simulink model "mavsim_chap10_6DOF"  (R2020b)
settings: Solver=ode15s  StartTime=0.0  StopTime=400  RelTol=1e-3  EnableMultiTasking=on
InitFcn:
  | param_chap10
undefined symbols (not defined in the file or in its folder): autopilot, drawPathError, Earth, forces_moments, js_decode_landing, js_encode_landing, P, path_follow, path_manager_chap10, sigbuilder_block, true_states, WGS84
libraries: simulink x7, simulink_extras x7, pid_lib x7, aerolibfltsims x2, instrumentlib x2, shared6dof x1, aerolibasang x1, aerolibtransform2 x1, aerolibanimutils x1, dspnetwork x1
(part 1 of 2)
settings Model: Creator=beard  LastModifiedBy=jk
settings DataIOCC: LimitDataPoints=on  SaveFormat=Array  SignalLoggingSaveFormat=ModelDataLogs  ReturnWorkspaceOutputs=off
settings OptimizationCC: ExpressionDepthLimit=2147483647  InitFltsAndDblsToZero=on  LifeSpan=inf
settings DebuggingCC: UnderspecifiedInitializationDetection=Classic  MergeDetectMultiDrivingBlocksExec=none  SolverPrmCheckMsg=warning  FcnCallInpInsideContextMsg=warning  StateNameClashWarn=warning  SFUnexpectedBacktrackingDiag=warning  SFNoUnconditionalDefaultTransitionDiag=warning  SFExecutionAtInitializationDiag=none  ArithmeticOperatorsInVariantConditions=warning
settings HardwareCC: ProdBitPerPointer=32  ProdBitPerSizeT=32  ProdBitPerPtrDiffT=32  ProdLargestAtomicFloat=None  ProdIntDivRoundTo=Undefined  ProdEndianess=Unspecified  ProdWordSize=32  ProdHWDeviceType=32-bit Generic
settings ModelReferenceCC: PropagateSignalLabelsOutOfModel=off
settings SFSimCC: SimUseLocalCustomCode=off  SimParseCustomCode=off  CustomCodeUndefinedFunction=UseInterfaceOnly
settings RTWCC: RTWUseLocalCustomCode=off
settings CodeAppCC: StateflowObjectComments=on
settings GRTTargetCC: TargetLangStandard=C89/C90 (ANSI)  CombineOutputUpdateFcns=off  GRTInterface=on
settings ConfigComp: CovMetricSettings=dw  CovSaveCumulativeToWorkspaceVar=on  CovSaveSingleToWorkspaceVar=on  CovExternalEMLEnable=off  CovSFcnEnable=off

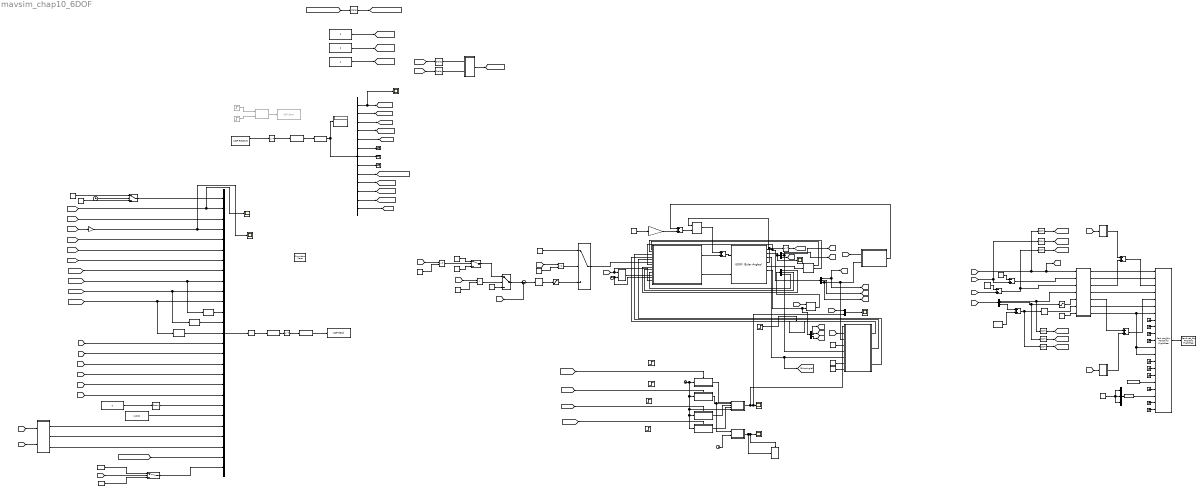
== system mavsim_chap10_6DOF ==
  note: 接受到来自航母终止盘旋指令
  note: 接受到来自航母的盘旋指令
  note: 开始着舰
  note: 开始降落
  note: 通过UDP接收数据，暂时通过自己创造Json的形式来测试是否正常接收，联调的时候将此区域内的发送部分删除只保留接收
  note: 发送部分用于测试使用
  note: 偏差XYZ
  note: 推力控制
  6DOF (Euler Angles) : shared6dof/6DOF (Euler Angles)  units=Metric (MKS)  mtype=Fixed  rep=Euler Angles  xme_0=[-5226.5 0 -600]  Vm_0=[80*cosd(-0) 0 80*sind(-0)]  eul_0=[0 -0*pi/180 0]  pm_0=[0 0 0]  mass_0=11000  mass_e=0.5  mass_f=2.0  inertia=[1000,0,0;0,2000,0;0,0,1000]  inertia_e=eye(3)  inertia_f=2*eye(3)  k_quat=1.0  vre_flag=on  abi_flag=off  aMode=0  xme_statename=''  Vm_statename=''  eul_statename=''  quat_statename=''  pm_statename=''  mass_statename=''
      settings: SourceProductBaseCode=AE,PW,MT,UV,VE,VP
  Add{,1,3..4,7} (5 alike) : Sum
  Add2 : Sum  Inputs=-+
  Add5 : Sum  Inputs=-+
  Clock{,1..3} (4 alike) : Clock
  Constant{,1,10,12,14,19..20} (7 alike) : Constant  Value=0
  Constant11 : Constant  Value=11000
  Constant13 : Constant  Value=2
  Constant{15..18,22} (5 alike) : Constant
  Constant2 : Constant  Value=-0.06
  Constant21 : Constant  Value=-40
  Constant3 : Constant  Value=3  OutDataTypeStr=uint32
  Constant4 : Constant  Value=-700
  Constant5 : Constant  Value=-300
  Constant6 : Constant  Value=80
  Constant7 : Constant  Value=120
  Constant8 : Constant  Value=70
  Constant9 : Constant  Value=-30
  Data Type Conversion : DataTypeConversion  OutDataTypeStr=double
  Data Type Conversion1 : DataTypeConversion  OutDataTypeStr=uint8
  Data Type Conversion2 : DataTypeConversion  OutDataTypeStr=single
  Delay : Delay  DelayLength=1  InitialCondition=0
  Demux{,1..2,4..5} (5 alike) : Demux  Outputs=3
  Demux3 : Demux  Outputs=13
  Discrete Derivative3 : simulink/Discrete/Discrete Derivative  gainval=1.0  ICPrevScaledInput=0.0  OutMin=[]  OutMax=[]  OutDataType=fixdt(1, 16)  OutScaling=2^-10  DoSatur=off
  Discrete Derivative4 : simulink/Discrete/Discrete Derivative  gainval=1.0  ICPrevScaledInput=0.0  OutMin=[]  OutMax=[]  OutDataType=fixdt(1, 16)  OutScaling=2^-10  DoSatur=off
  Discrete Derivative5 : simulink/Discrete/Discrete Derivative  gainval=1.0  ICPrevScaledInput=0.0  OutMin=[]  OutMax=[]  OutDataType=fixdt(1, 16)  OutScaling=2^-10  DoSatur=off
  Display : Display
  Force Moment : MATLAB Function  TreatAsAtomicUnit=on
  Gain : Gain  Gain=-1
  Gravitational acceleration : Constant  Value=9.81
  Gravitational acceleration1 : Constant  Value=-4/57.3
  Gravity in Earth Axes : Gain  Gain=[0; 0; 11000]  SaturateOnIntegerOverflow=on  OutDataTypeStr=Inherit: Same as input  ParamDataTypeStr=Inherit: Same as input
  GreaterThan : RelationalOperator  Operator=<=  OutDataTypeStr=boolean  RndMeth=Simplest
  GreaterThan1 : RelationalOperator  Operator=<  OutDataTypeStr=boolean  RndMeth=Simplest
  GreaterThan2 : RelationalOperator  OutDataTypeStr=boolean  RndMeth=Simplest
  Ground{,1..9} (10 alike) : Ground
  "Incidence, Sideslip, & Airspeed" : aerolibasang/Incidence, Sideslip, & Airspeed
  Interpreted MATLAB Function : MATLABFcn  MATLABFcn=js_decode_landing(u)
  Interpreted MATLAB Function1 : MATLABFcn  MATLABFcn=js_encode_landing(u)
  LLT : Subsystem
  LandingGear : MATLAB Function  TreatAsAtomicUnit=on
  MATLAB Function : MATLAB Function  TreatAsAtomicUnit=on
  MATLAB Function1 : MATLAB Function  TreatAsAtomicUnit=on
  MATLAB Function2 : MATLAB Function  Commented=on  TreatAsAtomicUnit=on
  MATLAB Function3 : MATLAB Function  TreatAsAtomicUnit=on
  Mux : Mux  Inputs=2
  Mux1 : Mux  Inputs=27
  Mux2 : Mux  Inputs=3
  PID Controller1 : pid_lib/PID Controller  Controller=PID  Form=Parallel  TimeDomain=Continuous-time  UseExternalTs=off  SampleTime=-1  IntegratorMethod=Forward Euler  FilterMethod=Forward Euler  ControllerParametersSource=internal  P=100000  I=5000  D=10  UseFilter=on  N=10/10  TunerSelectOption=Transfer Function Based (PID Tuner App)  InitialConditionSource=internal  InitialConditionForIntegrator=0  InitialConditionForFilter=0  DifferentiatorICPrevScaledInput=0  ExternalReset=none  TrackingMode=off  Kt=1  LimitOutput=off  SatLimitsSource=internal  UpperSaturationLimit=inf  LowerSaturationLimit=-inf  LinearizeAsGain=on  AntiWindupMode=none  Kb=1  POutMin=[]  POutMax=[]  IOutMin=[]  IOutMax=[]  DOutMin=[]  DOutMax=[]  NOutMin=[]  NOutMax=[]  SumOutMin=[]  SumOutMax=[]  SaturationOutMin=[]  SaturationOutMax=[]  PParamMin=[]  PParamMax=[]  IParamMin=[]  IParamMax=[]  DParamMin=[]  DParamMax=[]  NParamMin=[]  NParamMax=[]  KbParamMin=[]  KbParamMax=[]  KtParamMin=[]  KtParamMax=[]  KbOutMin=[]  KbOutMax=[]  KtOutMin=[]  KtOutMax=[]  IntegratorOutMin=[]  IntegratorOutMax=[]  FilterOutMin=[]  FilterOutMax=[]  SumI1OutMin=[]  SumI1OutMax=[]  SumI2OutMin=[]  SumI2OutMax=[]  SumI3OutMin=[]  SumI3OutMax=[]  SumI4OutMin=[]  SumI4OutMax=[]  SumDOutMin=[]  SumDOutMax=[]  DifferentiatorOutMin=[]  DifferentiatorOutMax=[]  FilterDiffOutCoefMin=[]  FilterDiffOutCoefMax=[]  ReciprocalOutMin=[]  ReciprocalOutMax=[]  SumDenOutMin=[]  SumDenOutMax=[]  SumNumOutMin=[]  SumNumOutMax=[]  DivideOutMin=[]  DivideOutMax=[]  UdiffTsProdOutMin=[]  UdiffTsProdOutMax=[]  NTsProdOutMin=[]  NTsProdOutMax=[]  UintegralTsProdOutMin=[]  UintegralTsProdOutMax=[]  UngainTsProdOutMin=[]  UngainTsProdOutMax=[]  IntegratorContinuousStateAttributes=''  IntegratorStateMustResolveToSignalObject=off  IntegratorRTWStateStorageClass=Auto  FilterContinuousStateAttributes=''  FilterStateMustResolveToSignalObject=off  FilterRTWStateStorageClass=Auto  ParallelPVariant=InternalParameters  IdealPVariant=Disabled  IVariant=InternalParameters  DVariant=InternalParameters  IntegratorVariant=Continuous  SatVariant=Disabled  AWVariant=Passthrough  PCopyVariant=Disabled  TRVariant=Disabled  FdbkBlocksVariant=Forward  IdealPFdbkVariant=Disabled  SatFdbkVariant=Disabled  DerivativeFilterVariant=ContFilter  NVariant=InternalParameters  NCopyVariant=Disabled  FilterICVariant=InternalICsFilter  IntegratorICVariant=InternalICs  ExternalResetVariant=Disabled  TRSumVariant=Passthrough  SumFdbkVariant=Disabled  SumVariant=Sum_PID  TsampFilterVariant=InternalTs  TsampNgainVariant=Passthrough  TsampIntegralVariant=Passthrough  ExternalSaturationOutDataTypeStr=Inherit: Same as second input
  Pack net_fdm Packet for FlightGear : aerolibfltsims/Pack net_fdm Packet for FlightGear  FlightGearVersion=v2.12  ShowPositionAttitudeInputs=on  ShowVelocityAccelerationInputs=off  ShowControlSurfacePositionInputs=on  ShowEngineFuelInputs=off  ShowLandingGearInputs=on  ShowEnvironmentInputs=off  SampleTime=1/30  packetVersion=24
      settings: SourceProductBaseCode=AE
  Product1 : Product  Multiplication=Matrix(*)
  Radians to Degrees : simulink_extras/Transformations/Radians to Degrees
  Ramp4 : simulink/Sources/Ramp  slope=-0.2  start=20  InitialOutput=1
  Saturation : Saturate  UpperLimit=40000  LowerLimit=0
  Saturation2 : Saturate  UpperLimit=20
  Scope{,1..6} (7 alike) : Scope
  Send net_fdm Packet to FlightGear : aerolibfltsims/Send net_fdm Packet to FlightGear  DestinationIpAddress=127.0.0.1  DestinationPort=5502  LocalIpPort=-1  varLen=off  SampleTime=1/30
      settings: SourceProductBaseCode=AE
  Signal1 : Step  Time=150  SampleTime=0
  Signal2 : Step  Time=165  SampleTime=0
  Signal5 : Step  Time=2  SampleTime=0
  Signal8 : Step  Time=20  SampleTime=0
  Simulation Pace : aerolibanimutils/Simulation Pace  SimulationPace=1  SleepMode=Auto  OutputPaceError=off  SampleTime=1
  Step : Step  After=2  SampleTime=0
  Subsystem : Subsystem
  Subsystem1 : Subsystem
  Subsystem2 : Subsystem
  Subsystem3 : Subsystem
  Subsystem4 : Subsystem
  Subsystem5 : Subsystem
  Subsystem7 : Subsystem
  Subsystem8 : Subsystem
  Subsystem9 : Subsystem
  Sum1 : Sum  Inputs=|+-
  Switch : Switch  Criteria=u2 > Threshold
  Switch1 : Switch  Criteria=u2 > Threshold
  Switch2 : Switch  Criteria=u2 > Threshold
  Switch4 : Switch  Criteria=u2 > Threshold  Threshold=5
  Switch5 : Switch  Criteria=u2 > Threshold  Threshold=0.01
  Terminator : Terminator
  Terminator1 : Terminator
  Terminator2 : Terminator
  To Wind Axes : Product  Multiplication=Matrix(*)  InputSameDT=on  SaturateOnIntegerOverflow=on  OutDataTypeStr=Inherit: Same as first input
  Transport Delay : TransportDelay  DelayTime=2
  Transport Delay1 : TransportDelay  DelayTime=2.5
  Transport Delay2 : TransportDelay  DelayTime=2.5
  Transport Delay3 : TransportDelay  DelayTime=2.5
  Transpose : Math  Operator=transpose  SaturateOnIntegerOverflow=on
  Transpose1 : Math  Operator=transpose  SignedPower=on  SaturateOnIntegerOverflow=on
  Transpose2 : Math  Operator=transpose  SaturateOnIntegerOverflow=on
  UDP Receive : dspnetwork/UDP Receive  localURL='0.0.0.0'  localPort=51002  remoteURL='192.168.3.238'  remotePort=-1  recvBufferSize=8192  dims=406  signalDatatype=uint8  isComplex=off  isVarSize=off  showBlockingTime=off  blockingTime=0  sampletime=0.01  blockPlatform=[]
  UDP Send : instrumentlib/UDP Send  Commented=on  Host=127.0.0.1  Port=51001  LocalPort=-1  EnablePortSharing=off  ByteOrder=BigEndian  OutputDatagramPacketSize=406  EnableBlockingMode=on  LocalAddress=127.0.0.1
  UDP Send1 : instrumentlib/UDP Send  Host=192.168.3.238  Port=51001  LocalPort=-1  EnablePortSharing=off  ByteOrder=BigEndian  OutputDatagramPacketSize=2000  EnableBlockingMode=on  LocalAddress=192.168.3.240
  Zero-Order Hold{,1..5} (6 alike) : ZeroOrderHold  SampleTime=-1
  jiaban1 : Subsystem
  jiaban2 : Subsystem
  landing : Step  Commented=on  Time=45  SampleTime=0.01
  start_landing : Step  Commented=on  Time=2  SampleTime=0.01
  wires:
  Clock2/1 -> Subsystem4/1(In1), Subsystem7/1(In1), Subsystem8/1(In1), MATLAB Function/5(time), Subsystem3/1(In1)
  Subsystem3/1(u) -> MATLAB Function/1(u)
  Subsystem4/1(u) -> MATLAB Function1/1(u), MATLAB Function/2(u1)
  MATLAB Function/1(y) -> Subsystem/1(CommandHeight), Mux/2, Scope3/1
  Clock/1 -> MATLAB Function1/2(time)
  Subsystem8/1(u) -> MATLAB Function/3(u2)
  Subsystem7/1(u) -> MATLAB Function/4(u3)
  MATLAB Function1/1(y) -> Subsystem5/1(Inport), Subsystem5/Enable, Scope2/1
  landing/1 -> MATLAB Function2/2(u2)
  MATLAB Function2/1(y) -> UDP Send/1
  Demux3/1 -> Scope4/1, [StartLanding]
  start_landing/1 -> MATLAB Function2/1(u1)
  UDP Receive/1 -> Transpose1/1
  Transpose1/1 -> Data Type Conversion/1
  Interpreted MATLAB Function/1 -> Demux3/1, Display/1
  Demux3/2 -> [StartTuning]
  Demux3/3 -> [StopTuning]
  Demux3/4 -> [Fault_FlapJam]
  Demux3/5 -> [Landing]
  Demux3/6 -> Terminator/1
  Demux3/7 -> Terminator1/1
  Demux3/8 -> Terminator2/1
  Demux3/9 -> [LandingGear_status_fromRhapsody]
  Demux3/13 -> [ReFly]
  Demux3/12 -> [Fault_Wind_z]
  Demux3/11 -> [Fault_Wind_y]
  Demux3/10 -> [Fault_Wind_x]
  Constant11/1 -> Mux1/22  "MassConfirm"
  Constant22/1 -> Switch5/3  "FinishLanding"
  Subsystem9/1(DeviationX) -> Mux1/23
  Discrete Derivative5/1 -> Mux1/14
  Transport Delay2/1 -> Mux1/21
  [carrier_Py] -> Discrete Derivative4/1, Mux1/10  "CarrierPosition_y"
  [X] -> Subsystem9/2(In2)
  Switch5/1 -> Mux1/27
  Delay/1 -> Interpreted MATLAB Function1/1
  [Vy] -> Mux1/16
  [q] -> Mux1/19
  [Vz] -> Mux1/17
  [r] -> Mux1/20
  Transpose2/1 -> Data Type Conversion1/1
  Clock3/1 -> Switch4/2
  [Z] -> Subsystem9/1(Trigger)
  [Vx] -> Mux1/15
  [p] -> Mux1/18
  [y] -> Mux1/3  "P_Ainfo_y"
  Constant20/1 -> Switch5/1  "FinishLanding"
  Subsystem9/3(DeviationZ) -> Mux1/25
  Constant14/1 -> Switch4/3
  [carrier_Px] -> Discrete Derivative3/1, Mux1/9  "CarrierPosition_x"
  Discrete Derivative3/1 -> Mux1/12
  Discrete Derivative4/1 -> Mux1/13
  Constant19/1 -> Transport Delay2/1  "HoldingPatternOff"
  [theta] -> Mux1/6  "P_Ainfo_theta"
  [carrier_Pz] -> Discrete Derivative5/1, Mux1/11  "CarrierPosition_z"
  Data Type Conversion1/1 -> UDP Send1/1
  Subsystem9/2(DeviationY) -> Mux1/24
  Gain/1 -> Scope5/1, Mux1/4  "P_Ainfo_z"
  [x] -> Scope6/1, Mux1/2  "P_Ainfo_x"
  Constant15/1 -> Switch4/1
  [phi] -> Mux1/5  "P_Ainfo_phi"
  [z] -> Gain/1
  Mux1/1 -> Delay/1
  Switch4/1 -> Mux1/1  "landingrRequest"
  [psi] -> Mux1/7  "P_Ainfo_psi"
  Interpreted MATLAB Function1/1 -> Transpose2/1
  [TuningStatus] -> Mux1/8  "TuningStatus"
  [LandingGear_status_toRhapsody] -> Mux1/26
  [Vx] -> Switch5/2
  Constant16/1 -> [carrier_Px]
  Constant17/1 -> [carrier_Py]
  Constant18/1 -> [carrier_Pz]
  [Z] -> GreaterThan1/1
  Demux4/2 -> [Vy]
  Demux2/3 -> [Z]
  [Z] -> Mux/1
  Demux5/3 -> [r]
  6DOF (Euler Angles)/1 -> Demux4/1, Force Moment/7(V)
  Add/1 -> 6DOF (Euler Angles)/1
  [StartLanding] -> Subsystem3/Trigger
  [Z] -> Subsystem/2(AcutalHeight)
  Constant/1 -> Subsystem/4(CommandYPosition)
  "Incidence, Sideslip, & Airspeed"/1 -> Force Moment/1(alpha)
  Demux5/2 -> [q]
  [Landing] -> Subsystem7/Trigger
  Transpose/1 -> [DCMeb]
  [Z] -> GreaterThan2/1
  [Z] -> Force Moment/13(z), Subsystem2/1(z)
  LandingGear/1(Fe) -> Add1/1
  "Incidence, Sideslip, & Airspeed"/2 -> Force Moment/2(beta)
  Switch2/1 -> Force Moment/6(T)
  Demux/2 -> Force Moment/9(q_B)
  Gravitational acceleration/1 -> Gravity in Earth Axes/1
  Demux2/1 -> [X]
  Constant2/1 -> Subsystem/8(CommandTheta)
  To Wind Axes/1 -> Add/1  "Fg"
  GreaterThan/1 -> Switch/2
  Demux2/2 -> [Y], Subsystem/5(AcutalYPosition)
  GreaterThan2/1 -> Switch2/2
  Clock1/1 -> Force Moment/12(time), Subsystem2/2(time)
  Demux/3 -> Force Moment/10(r_B)
  Sum1/1 -> PID Controller1/1
  6DOF (Euler Angles)/4 -> To Wind Axes/1, Transpose/1
  Gravity in Earth Axes/1 -> Add1/2
  Demux4/1 -> [Vx], [u]
  Product1/1 -> Demux/1
  Constant7/1 -> Switch/1
  [Z] -> GreaterThan/1
  Subsystem/2(Aileron) -> Force Moment/3(da)
  PID Controller1/1 -> Saturation/1
  Constant4/1 -> GreaterThan/2
  GreaterThan1/1 -> Switch1/2
  Subsystem/1(Elevator) -> Force Moment/4(de)
  Constant1/1 -> Subsystem/7(CommandPsi)
  Demux5/1 -> [p]
  Constant9/1 -> GreaterThan2/2
  Demux/1 -> Force Moment/8(p_B)
  Constant8/1 -> Switch1/3
  Switch/1 -> Switch1/1
  Step/1 -> Subsystem1/Enable
  Mux/1 -> Scope/1
  [Z] -> LandingGear/1(z)
  Demux4/3 -> [Vz], LandingGear/2(Vz), Subsystem/3(Vz)
  [u] -> Sum1/2
  Subsystem/3(Rudder) -> Force Moment/5(dr)
  Saturation/1 -> Switch2/3
  Constant5/1 -> GreaterThan1/2
  Switch1/1 -> Sum1/1
  Subsystem2/1(t) -> Force Moment/11(t)
  Constant6/1 -> Switch/3
  6DOF (Euler Angles)/3 -> [EulerAngle], Subsystem/6(EulerAngle)
  [DCMeb] -> Product1/1
  Force Moment/1(F) -> Add/2
  6DOF (Euler Angles)/2 -> Scope1/1, Demux2/1
  6DOF (Euler Angles)/5 -> "Incidence, Sideslip, & Airspeed"/1
  6DOF (Euler Angles)/6 -> Demux5/1, Product1/2
  Force Moment/2(M) -> 6DOF (Euler Angles)/2
  Constant10/1 -> Switch2/1
  Ground8/1 -> Pack net_fdm Packet for FlightGear/21
  Ground/1 -> Pack net_fdm Packet for FlightGear/8
  Add3/1 -> Pack net_fdm Packet for FlightGear/3
  Zero-Order Hold1/1 -> [y]
  Zero-Order Hold4/1 -> [theta]
  Demux1/3 -> Add7/1
  [Z] -> Add5/2
  Add5/1 -> Zero-Order Hold2/1, LLT/3(In3)
  Ground9/1 -> Pack net_fdm Packet for FlightGear/18
  Add2/1 -> LLT/2(In2)
  Constant21/1 -> Add2/1
  Ground3/1 -> Pack net_fdm Packet for FlightGear/11
  Zero-Order Hold/1 -> [x]
  Ground2/1 -> Pack net_fdm Packet for FlightGear/10
  Demux1/1 -> Zero-Order Hold3/1, LLT/4(In4)
  LLT/5(theta) -> Add4/1
  LLT/3(z) -> Add3/2
  LLT/6(psi) -> Pack net_fdm Packet for FlightGear/6
  Ground5/1 -> Pack net_fdm Packet for FlightGear/15
  Ground1/1 -> Pack net_fdm Packet for FlightGear/9
  Mux2/1 -> Data Type Conversion2/1
  LLT/7(angle) -> Pack net_fdm Packet for FlightGear/12, Pack net_fdm Packet for FlightGear/13, Pack net_fdm Packet for FlightGear/7
  Ground4/1 -> Pack net_fdm Packet for FlightGear/14
  Demux1/2 -> Zero-Order Hold4/1, Saturation2/1
  [Y] -> Add2/2, Zero-Order Hold1/1
  LLT/2(y) -> Pack net_fdm Packet for FlightGear/2
  Saturation2/1 -> LLT/5(In5)
  Constant12/1 -> LLT/7(In6)
  Constant13/1 -> Add5/1
  Zero-Order Hold2/1 -> [z]
  Radians to Degrees/1 -> LLT/6(In7)
  Add4/1 -> Pack net_fdm Packet for FlightGear/5
  LLT/4(phi) -> Pack net_fdm Packet for FlightGear/4
  Data Type Conversion2/1 -> Pack net_fdm Packet for FlightGear/19
  Ramp4/1 -> Mux2/3, Mux2/2, Mux2/1
  [EulerAngle] -> Demux1/1
  Pack net_fdm Packet for FlightGear/1 -> Send net_fdm Packet to FlightGear/1
  Constant3/1 -> Pack net_fdm Packet for FlightGear/17
  Ground7/1 -> Pack net_fdm Packet for FlightGear/20
  Zero-Order Hold3/1 -> [phi]
  Add7/1 -> Zero-Order Hold5/1, Radians to Degrees/1
  Zero-Order Hold5/1 -> [psi]
  jiaban1/1(Out1) -> Add3/1
  Gravitational acceleration1/1 -> Add7/2
  LLT/1(x) -> Pack net_fdm Packet for FlightGear/1
  [x1] -> jiaban2/1(In1)
  [x1] -> jiaban1/1(In1)
  [X] -> [x1], LLT/1(In1), Zero-Order Hold/1
  Ground6/1 -> Pack net_fdm Packet for FlightGear/16
  jiaban2/1(Out1) -> Add4/2
  [StartTuning] -> Subsystem4/Trigger
  [StopTuning] -> Subsystem8/Trigger
  [LandingGear_status_fromRhapsody] -> Transport Delay/1
  Transport Delay/1 -> [LandingGear_status_toRhapsody]
  Add1/1 -> To Wind Axes/2
  [StartTuning] -> Transport Delay1/1
  Transport Delay1/1 -> MATLAB Function3/1(u)
  [StopTuning] -> Transport Delay3/1
  Transport Delay3/1 -> MATLAB Function3/2(u1)
  MATLAB Function3/1(y) -> [TuningStatus]
  Data Type Conversion/1 -> Interpreted MATLAB Function/1

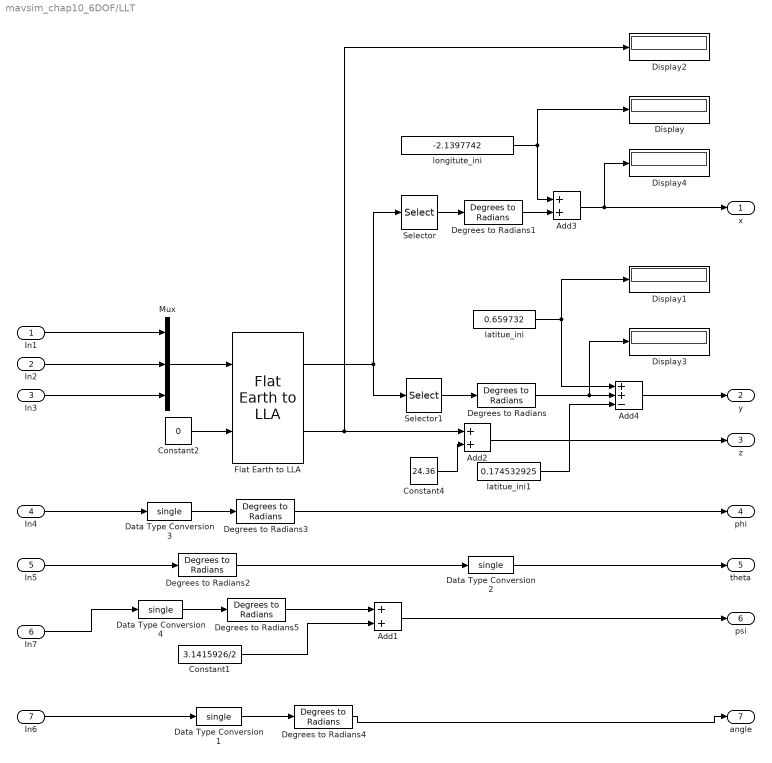
== system mavsim_chap10_6DOF/LLT ==
  In1 : Inport
  In2 : Inport  Port=2
  In3 : Inport  Port=3
  In4 : Inport  Port=4
  In5 : Inport  Port=5
  In7 : Inport  Port=6
  In6 : Inport  Port=7
  Add1 : Sum
  Add2 : Sum
  Add3 : Sum
  Add4 : Sum  Inputs=++-
  Constant1 : Constant  Value=3.1415926/2  OutDataTypeStr=single
  Constant2 : Constant  Value=0
  Constant4 : Constant  Value=24.36
  Data Type Conversion{1..4} (4 alike) : DataTypeConversion  OutDataTypeStr=single
  Degrees to Radians{,1..5} (6 alike) : simulink_extras/Transformations/Degrees to Radians
  Display{,1..4} (5 alike) : Display
  Flat Earth to LLA : aerolibtransform2/Flat Earth to LLA  units=Metric (MKS)  ptype=Earth (WGS84)  F=1/298.257223563  R=6378137  refPosPort=off  LL0=[0 10]  psi=0
  Mux : Mux  Inputs=3
  Selector : Selector  InputPortWidth=2  IndexOptions=Index vector (dialog)  Indices=[1]  OutputSizes=1
  Selector1 : Selector  InputPortWidth=2  IndexOptions=Index vector (dialog)  Indices=[2]  OutputSizes=1
  latitue_ini : Constant  Value=0.659732  OutDataTypeStr=double  LockScale=on
  latitue_ini1 : Constant  Value=0.174532925  OutDataTypeStr=double  LockScale=on
  longitute_ini : Constant  Value=-2.1397742  OutDataTypeStr=double  LockScale=on
  x : Outport
  y : Outport  Port=2
  z : Outport  Port=3
  phi : Outport  Port=4
  theta : Outport  Port=5
  psi : Outport  Port=6
  angle : Outport  Port=7
  wires:
  Degrees to Radians2/1 -> Data Type Conversion2/1
  Degrees to Radians4/1 -> angle/1
  Degrees to Radians1/1 -> Add3/2
  longitute_ini/1 -> Add3/1, Display/1
  In1/1 -> Mux/1
  In2/1 -> Mux/2
  Add3/1 -> x/1, Display4/1
  Flat Earth to LLA/2 -> Add2/1, Display2/1
  Data Type Conversion1/1 -> Degrees to Radians4/1
  latitue_ini/1 -> Add4/1, Display1/1
  Constant4/1 -> Add2/2
  Degrees to Radians/1 -> Add4/2, Display3/1
  latitue_ini1/1 -> Add4/3
  Add4/1 -> y/1
  Add2/1 -> z/1
  Selector1/1 -> Degrees to Radians/1
  Add1/1 -> psi/1
  Flat Earth to LLA/1 -> Selector1/1, Selector/1
  In4/1 -> Data Type Conversion3/1
  Constant1/1 -> Add1/2
  Constant2/1 -> Flat Earth to LLA/2
  In3/1 -> Mux/3
  Selector/1 -> Degrees to Radians1/1
  Mux/1 -> Flat Earth to LLA/1
  In6/1 -> Data Type Conversion1/1
  In5/1 -> Degrees to Radians2/1
  Data Type Conversion2/1 -> theta/1
  Data Type Conversion3/1 -> Degrees to Radians3/1
  Degrees to Radians3/1 -> phi/1
  In7/1 -> Data Type Conversion4/1
  Data Type Conversion4/1 -> Degrees to Radians5/1
  Degrees to Radians5/1 -> Add1/1

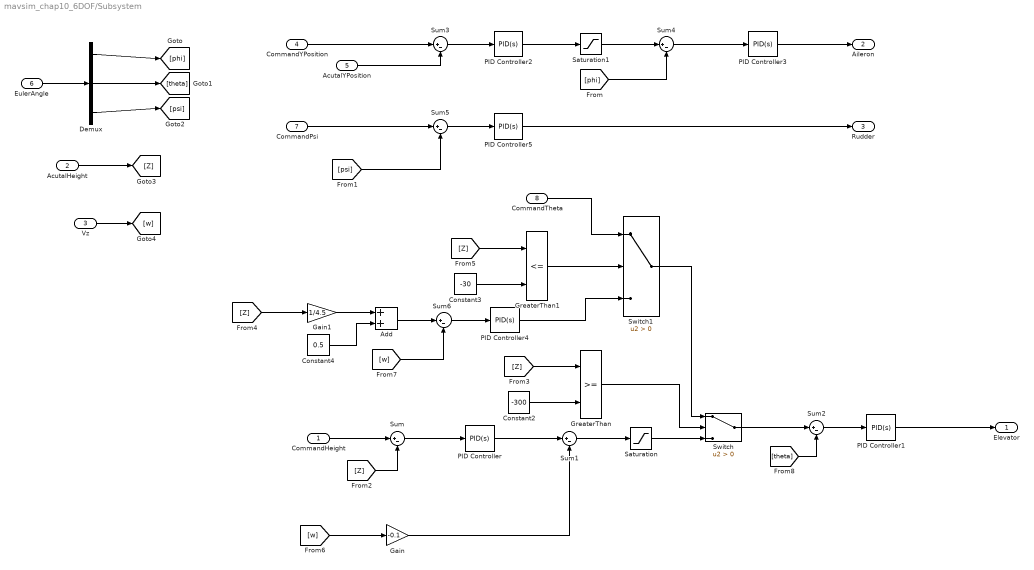
== system mavsim_chap10_6DOF/Subsystem ==
  CommandHeight : Inport
  AcutalHeight : Inport  Port=2
  Vz : Inport  Port=3
  CommandYPosition : Inport  Port=4
  AcutalYPosition : Inport  Port=5
  EulerAngle : Inport  Port=6
  CommandPsi : Inport  Port=7
  CommandTheta : Inport  Port=8
  Add : Sum
  Constant2 : Constant  Value=-300
  Constant3 : Constant  Value=-30
  Constant4 : Constant  Value=0.5
  Demux : Demux  Outputs=3
  Gain : Gain  Gain=-0.1
  Gain1 : Gain  Gain=1/4.5
  GreaterThan : RelationalOperator  OutDataTypeStr=boolean  RndMeth=Simplest
  GreaterThan1 : RelationalOperator  Operator=<=  OutDataTypeStr=boolean  RndMeth=Simplest
  PID Controller : pid_lib/PID Controller  Controller=PID  Form=Parallel  TimeDomain=Continuous-time  UseExternalTs=off  SampleTime=-1  IntegratorMethod=Forward Euler  FilterMethod=Forward Euler  ControllerParametersSource=internal  P=-0.5  I=-0.5/1000  D=-0.5*1000  UseFilter=on  N=1/1000  TunerSelectOption=Transfer Function Based (PID Tuner App)  InitialConditionSource=internal  InitialConditionForIntegrator=0  InitialConditionForFilter=0  DifferentiatorICPrevScaledInput=0  ExternalReset=none  TrackingMode=off  Kt=1  LimitOutput=off  SatLimitsSource=internal  UpperSaturationLimit=inf  LowerSaturationLimit=-inf  LinearizeAsGain=on  AntiWindupMode=none  Kb=1  POutMin=[]  POutMax=[]  IOutMin=[]  IOutMax=[]  DOutMin=[]  DOutMax=[]  NOutMin=[]  NOutMax=[]  SumOutMin=[]  SumOutMax=[]  SaturationOutMin=[]  SaturationOutMax=[]  PParamMin=[]  PParamMax=[]  IParamMin=[]  IParamMax=[]  DParamMin=[]  DParamMax=[]  NParamMin=[]  NParamMax=[]  KbParamMin=[]  KbParamMax=[]  KtParamMin=[]  KtParamMax=[]  KbOutMin=[]  KbOutMax=[]  KtOutMin=[]  KtOutMax=[]  IntegratorOutMin=[]  IntegratorOutMax=[]  FilterOutMin=[]  FilterOutMax=[]  SumI1OutMin=[]  SumI1OutMax=[]  SumI2OutMin=[]  SumI2OutMax=[]  SumI3OutMin=[]  SumI3OutMax=[]  SumI4OutMin=[]  SumI4OutMax=[]  SumDOutMin=[]  SumDOutMax=[]  DifferentiatorOutMin=[]  DifferentiatorOutMax=[]  FilterDiffOutCoefMin=[]  FilterDiffOutCoefMax=[]  ReciprocalOutMin=[]  ReciprocalOutMax=[]  SumDenOutMin=[]  SumDenOutMax=[]  SumNumOutMin=[]  SumNumOutMax=[]  DivideOutMin=[]  DivideOutMax=[]  UdiffTsProdOutMin=[]  UdiffTsProdOutMax=[]  NTsProdOutMin=[]  NTsProdOutMax=[]  UintegralTsProdOutMin=[]  UintegralTsProdOutMax=[]  UngainTsProdOutMin=[]  UngainTsProdOutMax=[]  IntegratorContinuousStateAttributes=''  IntegratorStateMustResolveToSignalObject=off  IntegratorRTWStateStorageClass=Auto  FilterContinuousStateAttributes=''  FilterStateMustResolveToSignalObject=off  FilterRTWStateStorageClass=Auto  ParallelPVariant=InternalParameters  IdealPVariant=Disabled  IVariant=InternalParameters  DVariant=InternalParameters  IntegratorVariant=Continuous  SatVariant=Disabled  AWVariant=Passthrough  PCopyVariant=Disabled  TRVariant=Disabled  FdbkBlocksVariant=Forward  IdealPFdbkVariant=Disabled  SatFdbkVariant=Disabled  DerivativeFilterVariant=ContFilter  NVariant=InternalParameters  NCopyVariant=Disabled  FilterICVariant=InternalICsFilter  IntegratorICVariant=InternalICs  ExternalResetVariant=Disabled  TRSumVariant=Passthrough  SumFdbkVariant=Disabled  SumVariant=Sum_PID  TsampFilterVariant=InternalTs  TsampNgainVariant=Passthrough  TsampIntegralVariant=Passthrough  ExternalSaturationOutDataTypeStr=Inherit: Same as second input
  PID Controller1 : pid_lib/PID Controller  Controller=PID  Form=Parallel  TimeDomain=Continuous-time  UseExternalTs=off  SampleTime=-1  IntegratorMethod=Forward Euler  FilterMethod=Forward Euler  ControllerParametersSource=internal  P=-100  I=-100/100  D=-100*100  UseFilter=on  N=1/100  TunerSelectOption=Transfer Function Based (PID Tuner App)  InitialConditionSource=internal  InitialConditionForIntegrator=0  InitialConditionForFilter=0  DifferentiatorICPrevScaledInput=0  ExternalReset=none  TrackingMode=off  Kt=1  LimitOutput=off  SatLimitsSource=internal  UpperSaturationLimit=inf  LowerSaturationLimit=-inf  LinearizeAsGain=on  AntiWindupMode=none  Kb=1  POutMin=[]  POutMax=[]  IOutMin=[]  IOutMax=[]  DOutMin=[]  DOutMax=[]  NOutMin=[]  NOutMax=[]  SumOutMin=[]  SumOutMax=[]  SaturationOutMin=[]  SaturationOutMax=[]  PParamMin=[]  PParamMax=[]  IParamMin=[]  IParamMax=[]  DParamMin=[]  DParamMax=[]  NParamMin=[]  NParamMax=[]  KbParamMin=[]  KbParamMax=[]  KtParamMin=[]  KtParamMax=[]  KbOutMin=[]  KbOutMax=[]  KtOutMin=[]  KtOutMax=[]  IntegratorOutMin=[]  IntegratorOutMax=[]  FilterOutMin=[]  FilterOutMax=[]  SumI1OutMin=[]  SumI1OutMax=[]  SumI2OutMin=[]  SumI2OutMax=[]  SumI3OutMin=[]  SumI3OutMax=[]  SumI4OutMin=[]  SumI4OutMax=[]  SumDOutMin=[]  SumDOutMax=[]  DifferentiatorOutMin=[]  DifferentiatorOutMax=[]  FilterDiffOutCoefMin=[]  FilterDiffOutCoefMax=[]  ReciprocalOutMin=[]  ReciprocalOutMax=[]  SumDenOutMin=[]  SumDenOutMax=[]  SumNumOutMin=[]  SumNumOutMax=[]  DivideOutMin=[]  DivideOutMax=[]  UdiffTsProdOutMin=[]  UdiffTsProdOutMax=[]  NTsProdOutMin=[]  NTsProdOutMax=[]  UintegralTsProdOutMin=[]  UintegralTsProdOutMax=[]  UngainTsProdOutMin=[]  UngainTsProdOutMax=[]  IntegratorContinuousStateAttributes=''  IntegratorStateMustResolveToSignalObject=off  IntegratorRTWStateStorageClass=Auto  FilterContinuousStateAttributes=''  FilterStateMustResolveToSignalObject=off  FilterRTWStateStorageClass=Auto  ParallelPVariant=InternalParameters  IdealPVariant=Disabled  IVariant=InternalParameters  DVariant=InternalParameters  IntegratorVariant=Continuous  SatVariant=Disabled  AWVariant=Passthrough  PCopyVariant=Disabled  TRVariant=Disabled  FdbkBlocksVariant=Forward  IdealPFdbkVariant=Disabled  SatFdbkVariant=Disabled  DerivativeFilterVariant=ContFilter  NVariant=InternalParameters  NCopyVariant=Disabled  FilterICVariant=InternalICsFilter  IntegratorICVariant=InternalICs  ExternalResetVariant=Disabled  TRSumVariant=Passthrough  SumFdbkVariant=Disabled  SumVariant=Sum_PID  TsampFilterVariant=InternalTs  TsampNgainVariant=Passthrough  TsampIntegralVariant=Passthrough  ExternalSaturationOutDataTypeStr=Inherit: Same as second input
  PID Controller2 : pid_lib/PID Controller  Controller=PID  Form=Parallel  TimeDomain=Continuous-time  UseExternalTs=off  SampleTime=-1  IntegratorMethod=Forward Euler  FilterMethod=Forward Euler  ControllerParametersSource=internal  P=0.005  I=0.005/10000  D=0.005*10000  UseFilter=on  N=1/10000  TunerSelectOption=Transfer Function Based (PID Tuner App)  InitialConditionSource=internal  InitialConditionForIntegrator=0  InitialConditionForFilter=0  DifferentiatorICPrevScaledInput=0  ExternalReset=none  TrackingMode=off  Kt=1  LimitOutput=off  SatLimitsSource=internal  UpperSaturationLimit=inf  LowerSaturationLimit=-inf  LinearizeAsGain=on  AntiWindupMode=none  Kb=1  POutMin=[]  POutMax=[]  IOutMin=[]  IOutMax=[]  DOutMin=[]  DOutMax=[]  NOutMin=[]  NOutMax=[]  SumOutMin=[]  SumOutMax=[]  SaturationOutMin=[]  SaturationOutMax=[]  PParamMin=[]  PParamMax=[]  IParamMin=[]  IParamMax=[]  DParamMin=[]  DParamMax=[]  NParamMin=[]  NParamMax=[]  KbParamMin=[]  KbParamMax=[]  KtParamMin=[]  KtParamMax=[]  KbOutMin=[]  KbOutMax=[]  KtOutMin=[]  KtOutMax=[]  IntegratorOutMin=[]  IntegratorOutMax=[]  FilterOutMin=[]  FilterOutMax=[]  SumI1OutMin=[]  SumI1OutMax=[]  SumI2OutMin=[]  SumI2OutMax=[]  SumI3OutMin=[]  SumI3OutMax=[]  SumI4OutMin=[]  SumI4OutMax=[]  SumDOutMin=[]  SumDOutMax=[]  DifferentiatorOutMin=[]  DifferentiatorOutMax=[]  FilterDiffOutCoefMin=[]  FilterDiffOutCoefMax=[]  ReciprocalOutMin=[]  ReciprocalOutMax=[]  SumDenOutMin=[]  SumDenOutMax=[]  SumNumOutMin=[]  SumNumOutMax=[]  DivideOutMin=[]  DivideOutMax=[]  UdiffTsProdOutMin=[]  UdiffTsProdOutMax=[]  NTsProdOutMin=[]  NTsProdOutMax=[]  UintegralTsProdOutMin=[]  UintegralTsProdOutMax=[]  UngainTsProdOutMin=[]  UngainTsProdOutMax=[]  IntegratorContinuousStateAttributes=''  IntegratorStateMustResolveToSignalObject=off  IntegratorRTWStateStorageClass=Auto  FilterContinuousStateAttributes=''  FilterStateMustResolveToSignalObject=off  FilterRTWStateStorageClass=Auto  ParallelPVariant=InternalParameters  IdealPVariant=Disabled  IVariant=InternalParameters  DVariant=InternalParameters  IntegratorVariant=Continuous  SatVariant=Disabled  AWVariant=Passthrough  PCopyVariant=Disabled  TRVariant=Disabled  FdbkBlocksVariant=Forward  IdealPFdbkVariant=Disabled  SatFdbkVariant=Disabled  DerivativeFilterVariant=ContFilter  NVariant=InternalParameters  NCopyVariant=Disabled  FilterICVariant=InternalICsFilter  IntegratorICVariant=InternalICs  ExternalResetVariant=Disabled  TRSumVariant=Passthrough  SumFdbkVariant=Disabled  SumVariant=Sum_PID  TsampFilterVariant=InternalTs  TsampNgainVariant=Passthrough  TsampIntegralVariant=Passthrough  ExternalSaturationOutDataTypeStr=Inherit: Same as second input
  PID Controller3 : pid_lib/PID Controller  Controller=PID  Form=Parallel  TimeDomain=Continuous-time  UseExternalTs=off  SampleTime=-1  IntegratorMethod=Forward Euler  FilterMethod=Forward Euler  ControllerParametersSource=internal  P=-20  I=-20/100  D=-20*100  UseFilter=on  N=1/100  TunerSelectOption=Transfer Function Based (PID Tuner App)  InitialConditionSource=internal  InitialConditionForIntegrator=0  InitialConditionForFilter=0  DifferentiatorICPrevScaledInput=0  ExternalReset=none  TrackingMode=off  Kt=1  LimitOutput=off  SatLimitsSource=internal  UpperSaturationLimit=inf  LowerSaturationLimit=-inf  LinearizeAsGain=on  AntiWindupMode=none  Kb=1  POutMin=[]  POutMax=[]  IOutMin=[]  IOutMax=[]  DOutMin=[]  DOutMax=[]  NOutMin=[]  NOutMax=[]  SumOutMin=[]  SumOutMax=[]  SaturationOutMin=[]  SaturationOutMax=[]  PParamMin=[]  PParamMax=[]  IParamMin=[]  IParamMax=[]  DParamMin=[]  DParamMax=[]  NParamMin=[]  NParamMax=[]  KbParamMin=[]  KbParamMax=[]  KtParamMin=[]  KtParamMax=[]  KbOutMin=[]  KbOutMax=[]  KtOutMin=[]  KtOutMax=[]  IntegratorOutMin=[]  IntegratorOutMax=[]  FilterOutMin=[]  FilterOutMax=[]  SumI1OutMin=[]  SumI1OutMax=[]  SumI2OutMin=[]  SumI2OutMax=[]  SumI3OutMin=[]  SumI3OutMax=[]  SumI4OutMin=[]  SumI4OutMax=[]  SumDOutMin=[]  SumDOutMax=[]  DifferentiatorOutMin=[]  DifferentiatorOutMax=[]  FilterDiffOutCoefMin=[]  FilterDiffOutCoefMax=[]  ReciprocalOutMin=[]  ReciprocalOutMax=[]  SumDenOutMin=[]  SumDenOutMax=[]  SumNumOutMin=[]  SumNumOutMax=[]  DivideOutMin=[]  DivideOutMax=[]  UdiffTsProdOutMin=[]  UdiffTsProdOutMax=[]  NTsProdOutMin=[]  NTsProdOutMax=[]  UintegralTsProdOutMin=[]  UintegralTsProdOutMax=[]  UngainTsProdOutMin=[]  UngainTsProdOutMax=[]  IntegratorContinuousStateAttributes=''  IntegratorStateMustResolveToSignalObject=off  IntegratorRTWStateStorageClass=Auto  FilterContinuousStateAttributes=''  FilterStateMustResolveToSignalObject=off  FilterRTWStateStorageClass=Auto  ParallelPVariant=InternalParameters  IdealPVariant=Disabled  IVariant=InternalParameters  DVariant=InternalParameters  IntegratorVariant=Continuous  SatVariant=Disabled  AWVariant=Passthrough  PCopyVariant=Disabled  TRVariant=Disabled  FdbkBlocksVariant=Forward  IdealPFdbkVariant=Disabled  SatFdbkVariant=Disabled  DerivativeFilterVariant=ContFilter  NVariant=InternalParameters  NCopyVariant=Disabled  FilterICVariant=InternalICsFilter  IntegratorICVariant=InternalICs  ExternalResetVariant=Disabled  TRSumVariant=Passthrough  SumFdbkVariant=Disabled  SumVariant=Sum_PID  TsampFilterVariant=InternalTs  TsampNgainVariant=Passthrough  TsampIntegralVariant=Passthrough  ExternalSaturationOutDataTypeStr=Inherit: Same as second input
  PID Controller4 : pid_lib/PID Controller  Controller=PID  Form=Parallel  TimeDomain=Continuous-time  UseExternalTs=off  SampleTime=-1  IntegratorMethod=Forward Euler  FilterMethod=Forward Euler  ControllerParametersSource=internal  P=-0.001  I=-0.001/1000  D=-0.001*100  UseFilter=on  N=1/100  TunerSelectOption=Transfer Function Based (PID Tuner App)  InitialConditionSource=internal  InitialConditionForIntegrator=0  InitialConditionForFilter=0  DifferentiatorICPrevScaledInput=0  ExternalReset=none  TrackingMode=off  Kt=1  LimitOutput=off  SatLimitsSource=internal  UpperSaturationLimit=inf  LowerSaturationLimit=-inf  LinearizeAsGain=on  AntiWindupMode=none  Kb=1  POutMin=[]  POutMax=[]  IOutMin=[]  IOutMax=[]  DOutMin=[]  DOutMax=[]  NOutMin=[]  NOutMax=[]  SumOutMin=[]  SumOutMax=[]  SaturationOutMin=[]  SaturationOutMax=[]  PParamMin=[]  PParamMax=[]  IParamMin=[]  IParamMax=[]  DParamMin=[]  DParamMax=[]  NParamMin=[]  NParamMax=[]  KbParamMin=[]  KbParamMax=[]  KtParamMin=[]  KtParamMax=[]  KbOutMin=[]  KbOutMax=[]  KtOutMin=[]  KtOutMax=[]  IntegratorOutMin=[]  IntegratorOutMax=[]  FilterOutMin=[]  FilterOutMax=[]  SumI1OutMin=[]  SumI1OutMax=[]  SumI2OutMin=[]  SumI2OutMax=[]  SumI3OutMin=[]  SumI3OutMax=[]  SumI4OutMin=[]  SumI4OutMax=[]  SumDOutMin=[]  SumDOutMax=[]  DifferentiatorOutMin=[]  DifferentiatorOutMax=[]  FilterDiffOutCoefMin=[]  FilterDiffOutCoefMax=[]  ReciprocalOutMin=[]  ReciprocalOutMax=[]  SumDenOutMin=[]  SumDenOutMax=[]  SumNumOutMin=[]  SumNumOutMax=[]  DivideOutMin=[]  DivideOutMax=[]  UdiffTsProdOutMin=[]  UdiffTsProdOutMax=[]  NTsProdOutMin=[]  NTsProdOutMax=[]  UintegralTsProdOutMin=[]  UintegralTsProdOutMax=[]  UngainTsProdOutMin=[]  UngainTsProdOutMax=[]  IntegratorContinuousStateAttributes=''  IntegratorStateMustResolveToSignalObject=off  IntegratorRTWStateStorageClass=Auto  FilterContinuousStateAttributes=''  FilterStateMustResolveToSignalObject=off  FilterRTWStateStorageClass=Auto  ParallelPVariant=InternalParameters  IdealPVariant=Disabled  IVariant=InternalParameters  DVariant=InternalParameters  IntegratorVariant=Continuous  SatVariant=Disabled  AWVariant=Passthrough  PCopyVariant=Disabled  TRVariant=Disabled  FdbkBlocksVariant=Forward  IdealPFdbkVariant=Disabled  SatFdbkVariant=Disabled  DerivativeFilterVariant=ContFilter  NVariant=InternalParameters  NCopyVariant=Disabled  FilterICVariant=InternalICsFilter  IntegratorICVariant=InternalICs  ExternalResetVariant=Disabled  TRSumVariant=Passthrough  SumFdbkVariant=Disabled  SumVariant=Sum_PID  TsampFilterVariant=InternalTs  TsampNgainVariant=Passthrough  TsampIntegralVariant=Passthrough  ExternalSaturationOutDataTypeStr=Inherit: Same as second input
  PID Controller5 : pid_lib/PID Controller  Controller=PID  Form=Parallel  TimeDomain=Continuous-time  UseExternalTs=off  SampleTime=-1  IntegratorMethod=Forward Euler  FilterMethod=Forward Euler  ControllerParametersSource=internal  P=-0.5  I=-0.5/1  D=-0.5*1  UseFilter=on  N=1/1  TunerSelectOption=Transfer Function Based (PID Tuner App)  InitialConditionSource=internal  InitialConditionForIntegrator=0  InitialConditionForFilter=0  DifferentiatorICPrevScaledInput=0  ExternalReset=none  TrackingMode=off  Kt=1  LimitOutput=off  SatLimitsSource=internal  UpperSaturationLimit=inf  LowerSaturationLimit=-inf  LinearizeAsGain=on  AntiWindupMode=none  Kb=1  POutMin=[]  POutMax=[]  IOutMin=[]  IOutMax=[]  DOutMin=[]  DOutMax=[]  NOutMin=[]  NOutMax=[]  SumOutMin=[]  SumOutMax=[]  SaturationOutMin=[]  SaturationOutMax=[]  PParamMin=[]  PParamMax=[]  IParamMin=[]  IParamMax=[]  DParamMin=[]  DParamMax=[]  NParamMin=[]  NParamMax=[]  KbParamMin=[]  KbParamMax=[]  KtParamMin=[]  KtParamMax=[]  KbOutMin=[]  KbOutMax=[]  KtOutMin=[]  KtOutMax=[]  IntegratorOutMin=[]  IntegratorOutMax=[]  FilterOutMin=[]  FilterOutMax=[]  SumI1OutMin=[]  SumI1OutMax=[]  SumI2OutMin=[]  SumI2OutMax=[]  SumI3OutMin=[]  SumI3OutMax=[]  SumI4OutMin=[]  SumI4OutMax=[]  SumDOutMin=[]  SumDOutMax=[]  DifferentiatorOutMin=[]  DifferentiatorOutMax=[]  FilterDiffOutCoefMin=[]  FilterDiffOutCoefMax=[]  ReciprocalOutMin=[]  ReciprocalOutMax=[]  SumDenOutMin=[]  SumDenOutMax=[]  SumNumOutMin=[]  SumNumOutMax=[]  DivideOutMin=[]  DivideOutMax=[]  UdiffTsProdOutMin=[]  UdiffTsProdOutMax=[]  NTsProdOutMin=[]  NTsProdOutMax=[]  UintegralTsProdOutMin=[]  UintegralTsProdOutMax=[]  UngainTsProdOutMin=[]  UngainTsProdOutMax=[]  IntegratorContinuousStateAttributes=''  IntegratorStateMustResolveToSignalObject=off  IntegratorRTWStateStorageClass=Auto  FilterContinuousStateAttributes=''  FilterStateMustResolveToSignalObject=off  FilterRTWStateStorageClass=Auto  ParallelPVariant=InternalParameters  IdealPVariant=Disabled  IVariant=InternalParameters  DVariant=InternalParameters  IntegratorVariant=Continuous  SatVariant=Disabled  AWVariant=Passthrough  PCopyVariant=Disabled  TRVariant=Disabled  FdbkBlocksVariant=Forward  IdealPFdbkVariant=Disabled  SatFdbkVariant=Disabled  DerivativeFilterVariant=ContFilter  NVariant=InternalParameters  NCopyVariant=Disabled  FilterICVariant=InternalICsFilter  IntegratorICVariant=InternalICs  ExternalResetVariant=Disabled  TRSumVariant=Passthrough  SumFdbkVariant=Disabled  SumVariant=Sum_PID  TsampFilterVariant=InternalTs  TsampNgainVariant=Passthrough  TsampIntegralVariant=Passthrough  ExternalSaturationOutDataTypeStr=Inherit: Same as second input
  Saturation : Saturate  UpperLimit=0.3  LowerLimit=-0.3
  Saturation1 : Saturate  UpperLimit=0.3  LowerLimit=-0.3
  Sum{,1..6} (7 alike) : Sum  Inputs=|+-
  Switch : Switch  Criteria=u2 > Threshold
  Switch1 : Switch  Criteria=u2 > Threshold
  Elevator : Outport
  Aileron : Outport  Port=2
  Rudder : Outport  Port=3
  wires:
  Sum/1 -> PID Controller/1
  Gain/1 -> Sum1/2
  Sum1/1 -> Saturation/1
  PID Controller/1 -> Sum1/1
  PID Controller1/1 -> Elevator/1
  Sum2/1 -> PID Controller1/1
  [theta] -> Sum2/2
  [w] -> Gain/1
  CommandHeight/1 -> Sum/1
  CommandYPosition/1 -> Sum3/1
  AcutalYPosition/1 -> Sum3/2
  Sum3/1 -> PID Controller2/1
  PID Controller2/1 -> Saturation1/1
  Saturation1/1 -> Sum4/1
  EulerAngle/1 -> Demux/1
  Demux/1 -> [phi]
  Demux/2 -> [theta]
  Demux/3 -> [psi]
  [phi] -> Sum4/2
  Sum4/1 -> PID Controller3/1
  PID Controller3/1 -> Aileron/1
  CommandPsi/1 -> Sum5/1
  [psi] -> Sum5/2
  Sum5/1 -> PID Controller5/1
  PID Controller5/1 -> Rudder/1
  Saturation/1 -> Switch/3
  AcutalHeight/1 -> [Z]
  [Z] -> Sum/2
  [Z] -> GreaterThan/1
  Constant2/1 -> GreaterThan/2
  GreaterThan/1 -> Switch/2
  Switch1/1 -> Switch/1
  Constant3/1 -> GreaterThan1/2
  [Z] -> GreaterThan1/1
  GreaterThan1/1 -> Switch1/2
  [Z] -> Gain1/1
  Gain1/1 -> Add/1
  Constant4/1 -> Add/2
  Add/1 -> Sum6/1
  Vz/1 -> [w]
  [w] -> Sum6/2
  Sum6/1 -> PID Controller4/1
  PID Controller4/1 -> Switch1/3
  CommandTheta/1 -> Switch1/1
  Switch/1 -> Sum2/1

== system mavsim_chap10_6DOF/Subsystem1 ==
  Enable : EnablePort
  Signal Builder2 : Subsystem  Tag=STV Subsys  LoadFcn=sigbuilder_block('load');  StartFcn=sigbuilder_block('start');  StopFcn=sigbuilder_block('stop');  ClipboardFcn=sigbuilder_block('clipboard');  mask(Sigbuilder block){tuvar=[0:10]}
      mask help: Simulink:masks:SigbuilderBlock_MD
      mask init:
      | if ~strcmp(get_param(bdroot(gcbh),'SimulationStatus'),'stopped') tuvar = sigbuilder_block('maskInit'); end
      settings: CopyFcn=sigbuilder_block('copy');  DeleteFcn=sigbuilder_block('delete');  ModelCloseFcn=sigbuilder_block('modelClose');  PreSaveFcn=sigbuilder_block('preSave');  PauseFcn=sigbuilder_block('pause');  ContinueFcn=sigbuilder_block('continue');  NameChangeFcn=sigbuilder_block('namechange');  OpenFcn=sigbuilder_block('open',[9.6 245.4 460.2 318.6 ]);  CloseFcn=sigbuilder_block('close');
      mask Display: plot(0, 0, 100, 100,[2, 2, 32, 32, 2], [68, 8, 8, 68, 68],[32, 2], [38, 38], [32, 19, 2],[53, 60, 44], [32, 17, 17, 2],[16, 16, 31, 31]);txt = getActiveGroup(gcbh);text(2, 100, txt,'verticalAlignment', 'top');
  Signal 1 : Outport  InitialOutput=-600
  wires:
  Signal Builder2/1(Signal 1) -> Signal 1/1

== system mavsim_chap10_6DOF/Subsystem2 ==
  z : Inport
  time : Inport  Port=2
  Constant : Constant
  Constant1 : Constant  Value=0
  Subsystem1 : Subsystem
  Switch : Switch  Threshold=-1
  t : Outport
  wires:
  time/1 -> Subsystem1/1(In1)
  Subsystem1/1(Out1) -> t/1
  z/1 -> Switch/2
  Constant/1 -> Switch/1
  Constant1/1 -> Switch/3
  Switch/1 -> Subsystem1/Trigger

== system mavsim_chap10_6DOF/Subsystem3 ==
  In1 : Inport
  Trigger : TriggerPort  VariantControl=Variant  PortDimensions=1
  u : Outport
  wires:
  In1/1 -> u/1

== system mavsim_chap10_6DOF/Subsystem4 ==
  In1 : Inport
  Trigger : TriggerPort  VariantControl=Variant  PortDimensions=1
  u : Outport
  wires:
  In1/1 -> u/1

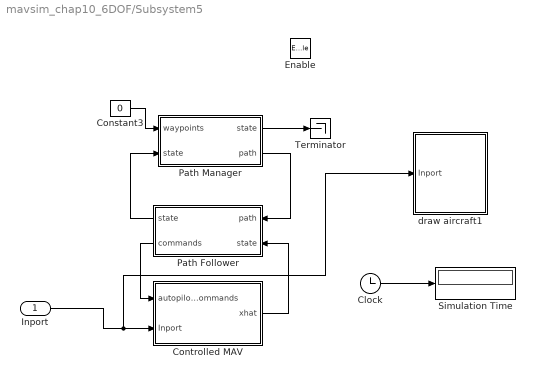
== system mavsim_chap10_6DOF/Subsystem5 ==
  Inport : Inport
  Enable : EnablePort
  Clock : Clock
  Constant3 : Constant  Value=0
  Controlled MAV : Subsystem
      mask Display: image(imread('batcam.png'))
  Path Follower : Subsystem
  Path Manager : Subsystem
  Simulation Time : Display
  Terminator : Terminator
  draw aircraft1 : Subsystem
      mask Display: image(imread('tv.jpg'))
  wires:
  Controlled MAV/1(xhat) -> Path Follower/2(state)
  Constant3/1 -> Path Manager/1(waypoints)
  Path Follower/2(commands) -> Controlled MAV/1(autopilot commands)
  Path Follower/1("state ") -> Path Manager/2(state)
  Clock/1 -> Simulation Time/1
  Path Manager/2(path) -> Path Follower/1(path)
  Path Manager/1("state ") -> Terminator/1
  Inport/1 -> draw aircraft1/1(Inport), Controlled MAV/2(Inport)

== system mavsim_chap10_6DOF/Subsystem7 ==
  In1 : Inport
  Trigger : TriggerPort  VariantControl=Variant  PortDimensions=1
  u : Outport
  wires:
  In1/1 -> u/1

== system mavsim_chap10_6DOF/Subsystem8 ==
  In1 : Inport
  Trigger : TriggerPort  VariantControl=Variant  PortDimensions=1
  u : Outport
  wires:
  In1/1 -> u/1

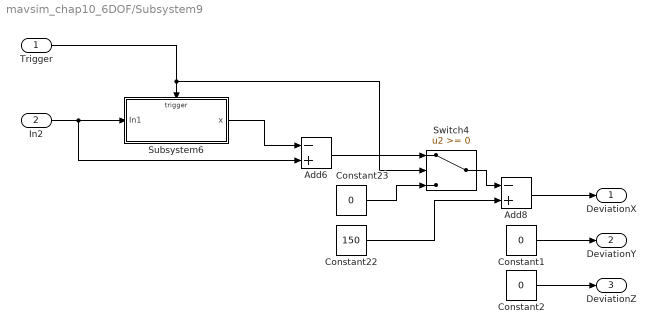
== system mavsim_chap10_6DOF/Subsystem9 ==
  Trigger : Inport
  In2 : Inport  Port=2
  Add6 : Sum  Inputs=-+
  Add8 : Sum  Inputs=-+
  Constant1 : Constant  Value=0
  Constant2 : Constant  Value=0
  Constant22 : Constant  Value=150
  Constant23 : Constant  Value=0
  Subsystem6 : Subsystem
  Switch4 : Switch
  DeviationX : Outport
  DeviationY : Outport  Port=2
  DeviationZ : Outport  Port=3
  wires:
  Trigger/1 -> Switch4/2, Subsystem6/Trigger
  In2/1 -> Add6/2, Subsystem6/1(In1)
  Add6/1 -> Switch4/1
  Constant22/1 -> Add8/2
  Subsystem6/1(x) -> Add6/1
  Add8/1 -> DeviationX/1
  Constant23/1 -> Switch4/3
  Switch4/1 -> Add8/1
  Constant1/1 -> DeviationY/1
  Constant2/1 -> DeviationZ/1

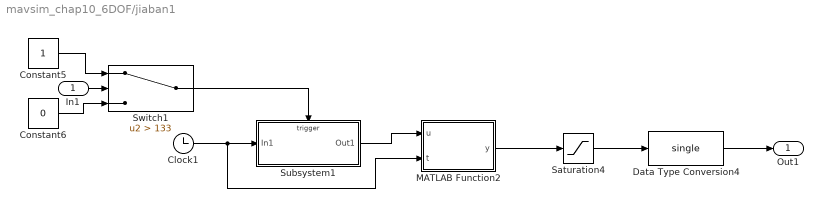
== system mavsim_chap10_6DOF/jiaban1 ==
  In1 : Inport
  Clock1 : Clock
  Constant5 : Constant
  Constant6 : Constant  Value=0
  Data Type Conversion4 : DataTypeConversion  OutDataTypeStr=single
  MATLAB Function2 : MATLAB Function  TreatAsAtomicUnit=on
  Saturation4 : Saturate  UpperLimit=20
  Subsystem1 : Subsystem
  Switch1 : Switch  Criteria=u2 > Threshold  Threshold=133
  Out1 : Outport
  wires:
  MATLAB Function2/1(y) -> Saturation4/1
  Clock1/1 -> MATLAB Function2/2(t), Subsystem1/1(In1)
  Constant5/1 -> Switch1/1
  Switch1/1 -> Subsystem1/Trigger
  In1/1 -> Switch1/2
  Saturation4/1 -> Data Type Conversion4/1
  Subsystem1/1(Out1) -> MATLAB Function2/1(u)
  Constant6/1 -> Switch1/3
  Data Type Conversion4/1 -> Out1/1

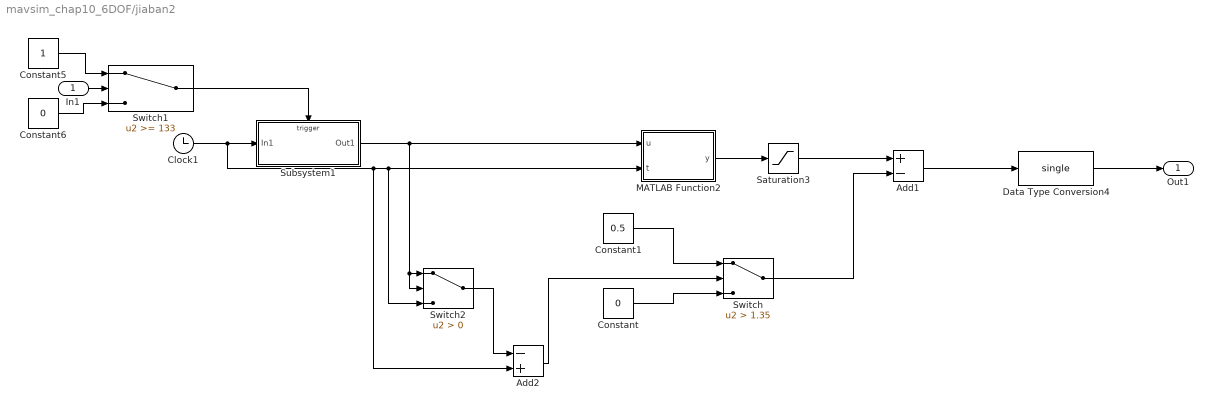
== system mavsim_chap10_6DOF/jiaban2 ==
  In1 : Inport
  Add1 : Sum  Inputs=+-
  Add2 : Sum  Inputs=-+
  Clock1 : Clock
  Constant : Constant  Value=0
  Constant1 : Constant  Value=0.5
  Constant5 : Constant
  Constant6 : Constant  Value=0
  Data Type Conversion4 : DataTypeConversion  OutDataTypeStr=single
  MATLAB Function2 : MATLAB Function  TreatAsAtomicUnit=on
  Saturation3 : Saturate
  Subsystem1 : Subsystem
  Switch : Switch  Criteria=u2 > Threshold  Threshold=1.35
  Switch1 : Switch  Threshold=133
  Switch2 : Switch  Criteria=u2 > Threshold
  Out1 : Outport
  wires:
  Constant6/1 -> Switch1/3
  Subsystem1/1(Out1) -> Switch2/1, Switch2/2, MATLAB Function2/1(u)
  In1/1 -> Switch1/2
  Switch1/1 -> Subsystem1/Trigger
  Constant5/1 -> Switch1/1
  Clock1/1 -> Subsystem1/1(In1), Add2/2, Switch2/3, MATLAB Function2/2(t)
  MATLAB Function2/1(y) -> Saturation3/1
  Constant/1 -> Switch/3
  Constant1/1 -> Switch/1
  Switch/1 -> Add1/2
  Saturation3/1 -> Add1/1
  Add1/1 -> Data Type Conversion4/1
  Data Type Conversion4/1 -> Out1/1
  Switch2/1 -> Add2/1
  Add2/1 -> Switch/2

== system mavsim_chap10_6DOF/Subsystem1/Signal Builder2 ==
  Demux : Demux  Tag=STV Demux  Outputs=1
      settings: DisplayOption=none
  FromWs : FromWorkspace  Tag=STV FromWs  VariableName=tuvar
      SigBuilderData=|
      | common.afterFinalStr = 'Extrapolate'
      | common.sampleTime = 0
      | dataSet.timeRange = [0 100]
      | dataSet.name = 'Group 1'
      | sbobj.Groups.Name = 'Group 1'
      | sbobj.Groups.Signals.Name = 'Signal 1'
      | sbobj.Groups.Signals.XData = [0 2 3 50 64 100]
      | sbobj.Groups.Signals.YData = [-600 -600 -600 -290 0 0]
      | sbobj.Groups.TimeRange = [0 100]
  Signal 1 : Outport  Tag=STV Outport
  wires:
  Demux/1 -> Signal 1/1
  FromWs/1 -> Demux/1

== system mavsim_chap10_6DOF/Subsystem2/Subsystem1 ==
  In1 : Inport
  Trigger : TriggerPort  VariantControl=Variant  PortDimensions=1
  Out1 : Outport  InitialOutput=100
  wires:
  In1/1 -> Out1/1

== system mavsim_chap10_6DOF/Subsystem5/Controlled MAV ==
  note: sensors
  note: control surfaces
      | commands
  autopilot commands : Inport
  Inport : Inport  Port=2
  Autopilot : Subsystem
      mask Display: image(imread('kestrel.jpg'))
  MAV1 : Subsystem
      mask Display: image(imread('batcam.png'))
  Memory : Memory
  Wind1 : Subsystem
  xhat : Outport
  wires:
  Wind1/1(Wind) -> MAV1/2(wind)
  Autopilot/2(delta) -> MAV1/1(delta)
  autopilot commands/1 -> Autopilot/1(commands)
  Autopilot/1(xhat) -> Memory/1
  Memory/1 -> xhat/1
  MAV1/1(x) -> Autopilot/2(x)
  Inport/1 -> Autopilot/3(Inport)

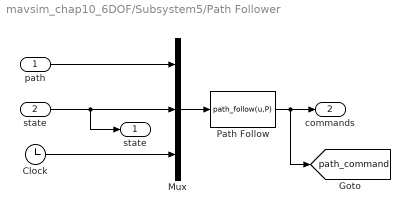
== system mavsim_chap10_6DOF/Subsystem5/Path Follower ==
  path : Inport
  state : Inport  Port=2
  Clock : Clock
  Mux : Mux  Inputs=3
  Path Follow : MATLABFcn  MATLABFcn=path_follow(u,P)  OutputDimensions=3  SampleTime=P.Ts
  "state " : Outport
  commands : Outport  Port=2
  tag scope: path_command=global
  wires:
  Path Follow/1 -> commands/1, [path_command]
  Mux/1 -> Path Follow/1
  path/1 -> Mux/1
  Clock/1 -> Mux/3
  state/1 -> Mux/2, "state "/1

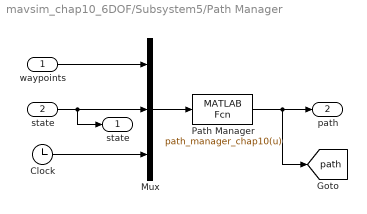
== system mavsim_chap10_6DOF/Subsystem5/Path Manager ==
  waypoints : Inport
  state : Inport  Port=2
  Clock : Clock
  Mux : Mux  Inputs=3
  Path Manager : MATLABFcn  MATLABFcn=path_manager_chap10(u)  OutputDimensions=13  SampleTime=P.Ts
  "state " : Outport
  path : Outport  Port=2
  tag scope: path=global
  wires:
  Path Manager/1 -> path/1, [path]
  Mux/1 -> Path Manager/1
  Clock/1 -> Mux/3
  state/1 -> Mux/2, "state "/1
  waypoints/1 -> Mux/1

== system mavsim_chap10_6DOF/Subsystem5/draw aircraft1 ==
  Inport : Inport
  Clock2 : Clock
  Mux : Mux  Inputs=3
  Sum : Sum  Inputs=|+-
  drawPathError : MATLABFcn  MATLABFcn=drawPathError(u)  OutputDimensions=0  SampleTime=0.1
  wires:
  [state] -> Mux/1
  Mux/1 -> drawPathError/1
  [path] -> Mux/3
  Inport/1 -> Sum/2
  Sum/1 -> Mux/2
  Clock2/1 -> Sum/1

== system mavsim_chap10_6DOF/Subsystem9/Subsystem6 ==
  In1 : Inport
  Trigger : TriggerPort  VariantControl=Variant  PortDimensions=1
  x : Outport  InitialOutput=0
  wires:
  In1/1 -> x/1

== system mavsim_chap10_6DOF/jiaban1/Subsystem1 ==
  In1 : Inport
  Trigger : TriggerPort  VariantControl=Variant  PortDimensions=1
  Out1 : Outport
  wires:
  In1/1 -> Out1/1

== system mavsim_chap10_6DOF/jiaban2/Subsystem1 ==
  In1 : Inport
  Trigger : TriggerPort  VariantControl=Variant  PortDimensions=1
  Out1 : Outport
  wires:
  In1/1 -> Out1/1

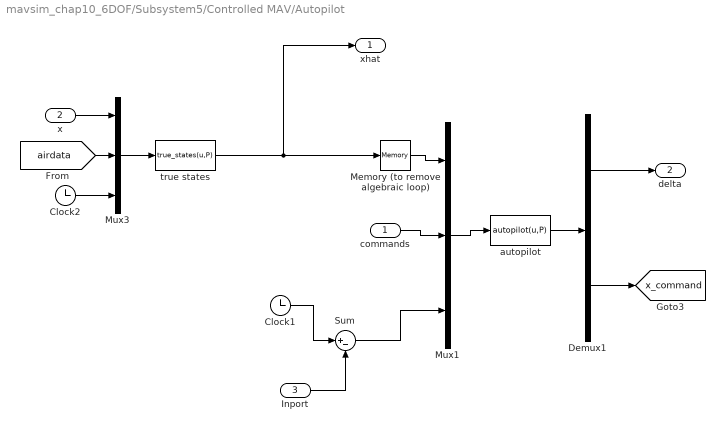
== system mavsim_chap10_6DOF/Subsystem5/Controlled MAV/Autopilot ==
  commands : Inport
  x : Inport  Port=2
  Inport : Inport  Port=3
  Clock1 : Clock
  Clock2 : Clock
  Demux1 : Demux  Outputs=[4;12]
  Memory (to remove algebraic loop) : Memory
  Mux1 : Mux  Inputs=3
  Mux3 : Mux  Inputs=3
  Sum : Sum  Inputs=|+-
  autopilot : MATLABFcn  MATLABFcn=autopilot(u,P)  OutputDimensions=4+12  SampleTime=P.Ts
  true states : MATLABFcn  MATLABFcn=true_states(u,P)  OutputDimensions=19  SampleTime=P.Ts
  xhat : Outport
  delta : Outport  Port=2
  tag scope: x_command=global
  wires:
  Mux1/1 -> autopilot/1
  autopilot/1 -> Demux1/1
  Demux1/1 -> delta/1
  Demux1/2 -> [x_command]
  commands/1 -> Mux1/2
  Memory (to remove algebraic loop)/1 -> Mux1/1
  Mux3/1 -> true states/1
  [airdata] -> Mux3/2
  Clock2/1 -> Mux3/3
  true states/1 -> xhat/1, Memory (to remove algebraic loop)/1
  x/1 -> Mux3/1
  Clock1/1 -> Sum/1
  Sum/1 -> Mux1/3
  Inport/1 -> Sum/2

== system mavsim_chap10_6DOF/Subsystem5/Controlled MAV/MAV1 ==
  note: Forces & Moments
  note: States
  delta : Inport
  wind : Inport  Port=2
  Dynamics : S-Function  FunctionName=mav_dynamics  Parameters=P  SFunctionDeploymentMode=off  EnableBusSupport=off
  Forces & Moments : Subsystem
  x : Outport
  tag scope: airdata=global, state=global
  wires:
  Dynamics/1 -> x/1, Forces & Moments/1(x), [state]
  Forces & Moments/1("[F M]") -> Dynamics/1
  Forces & Moments/2(air data) -> [airdata]
  delta/1 -> Forces & Moments/2(delta)
  wind/1 -> Forces & Moments/3(wind)
